simulink model "oving2"  (R2023a)
settings: Solver=ode1  StartTime=0.0  StopTime=25  FixedStep=0.01  RelTol=1e-9  AbsTol=1e-9
values from neighbouring files (symbols this model uses):
  a = input('Skriv inn tallet "a" mellom 0 og 10: ')    [kap2_matlab_kode.m]    (also in kap3_kode_for_alle_figurene.m = 3)
  b = input('Skriv inn tallet "b" mellom 0 og 10: ')    [kap2_matlab_kode.m]
  c = 3    [kap2_matlab_kode.m]    (also in kap3_kode_for_alle_figurene.m = 0.785398163397)
  d = 6.4    [kap2_matlab_kode.m]    (also in kap3_kode_for_alle_figurene.m = 4)
  f = int8(d)    [kap2_matlab_kode.m]    (also in kap3_kode_for_alle_figurene.m = sin(t); oving3_LL.m = 4.2)
  g = 5    [kap2_matlab_kode.m]
  h = 3    [kap2_matlab_kode.m]
  k = length(x)    [kap2_matlab_kode.m]    (also in kap3_kode_for_alle_figurene.m = 2; oving3_LL.m = 2)
  n = 7    [oving3_LL.m]
undefined symbols (not defined in the file or in its folder): i, j, l, m, o, p
libraries: simulink x16
settings Model: Creator=tormod  LastModifiedBy=redfox
settings DebuggingCC: UnconnectedInputMsg=warning  UnconnectedOutputMsg=warning  UnconnectedLineMsg=warning
settings ModelReferenceCC: EnableRefExpFcnMdlSchedulingChecks=on
settings RTWCC: DLArmComputeVersion=19.05

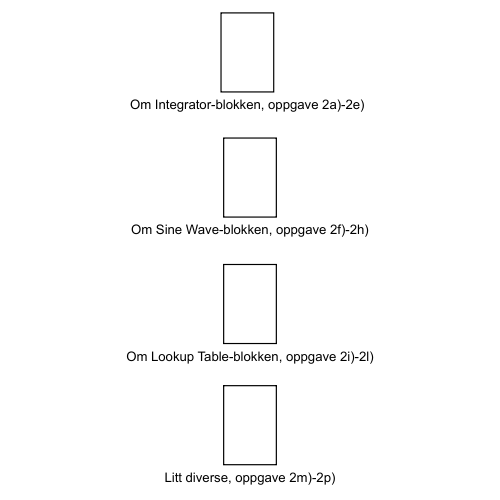
[thumbnail: Simulink's stored preview of the top-level diagram]
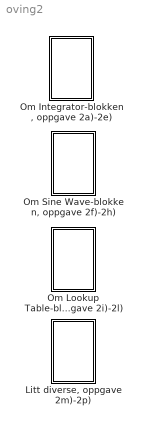
== system oving2 ==
  "Litt diverse, oppgave 2m)-2p)" : Subsystem
  "Om Integrator-blokken, oppgave 2a)-2e)" : Subsystem
  "Om Lookup Table-blokken, oppgave 2i)-2l)" : Subsystem
  "Om Sine Wave-blokken, oppgave 2f)-2h)" : Subsystem

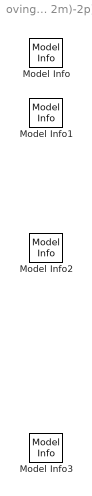
== system oving2/Litt diverse, oppgave 2m)-2p) ==
  Model Info : simulink/Model-Wide Utilities/Model Info  Frame=on  DisplayStringWithTags=m)  HorizontalTextAlignment=Center  LeftAlignmentValue=0.5
  Model Info1 : simulink/Model-Wide Utilities/Model Info  Frame=on  DisplayStringWithTags=n)  HorizontalTextAlignment=Center  LeftAlignmentValue=0.5
  Model Info2 : simulink/Model-Wide Utilities/Model Info  Frame=on  DisplayStringWithTags=o)  HorizontalTextAlignment=Center  LeftAlignmentValue=0.5
  Model Info3 : simulink/Model-Wide Utilities/Model Info  Frame=on  DisplayStringWithTags=p)  HorizontalTextAlignment=Center  LeftAlignmentValue=0.5

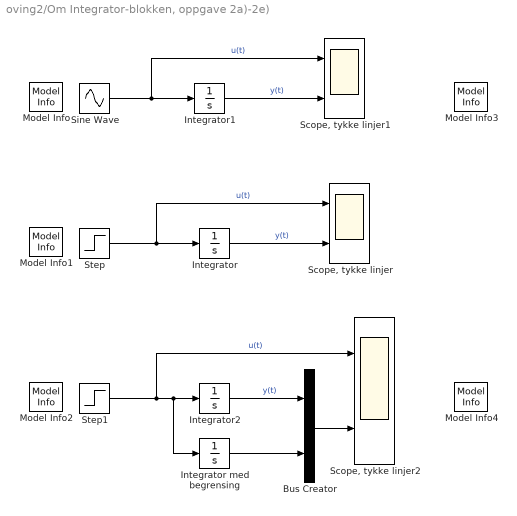
== system oving2/Om Integrator-blokken, oppgave 2a)-2e) ==
  Bus Creator : BusCreator  Inputs=2
  Integrator : Integrator  InitialCondition=-20
      settings: AttributesFormatString=IC = %<InitialCondition>
  Integrator med begrensing : Integrator  InitialCondition=-20  LimitOutput=on  UpperSaturationLimit=30
      settings: AttributesFormatString=|
      | IC = %<InitialCondition>
      | Max = %<UpperSaturationLimit>
      | Min = %<LowerSaturationLimit>
  Integrator1 : Integrator
      settings: AttributesFormatString=IC = %<InitialCondition>
  Integrator2 : Integrator  InitialCondition=-20
      settings: AttributesFormatString=IC = %<InitialCondition>
  Model Info : simulink/Model-Wide Utilities/Model Info  Frame=on  DisplayStringWithTags=a)  HorizontalTextAlignment=Center  LeftAlignmentValue=0.5
  Model Info1 : simulink/Model-Wide Utilities/Model Info  Frame=on  DisplayStringWithTags=b)  HorizontalTextAlignment=Center  LeftAlignmentValue=0.5
  Model Info2 : simulink/Model-Wide Utilities/Model Info  Frame=on  DisplayStringWithTags=c)  HorizontalTextAlignment=Center  LeftAlignmentValue=0.5
  Model Info3 : simulink/Model-Wide Utilities/Model Info  Frame=on  DisplayStringWithTags=d)  HorizontalTextAlignment=Center  LeftAlignmentValue=0.5
  Model Info4 : simulink/Model-Wide Utilities/Model Info  Frame=on  DisplayStringWithTags=e)  HorizontalTextAlignment=Center  LeftAlignmentValue=0.5
  "Scope, tykke linjer" : Scope  NumInputPorts=2
  "Scope, tykke linjer1" : Scope  NumInputPorts=2
  "Scope, tykke linjer2" : Scope  NumInputPorts=2
  Sine Wave : Sin  Amplitude=2  Frequency=5  SampleTime=0
      settings: AttributesFormatString=u(t) = %<Amplitude> sin(%<Frequency>t + %<Phase>) + %<Bias>
  Step : Step  Time=5  After=4  SampleTime=0
      settings: AttributesFormatString=|
      | u(t) = %<Before> for t < %<Time>s
      |       = %<After> for t > %<Time>s
  Step1 : Step  Time=5  After=4  SampleTime=0
      settings: AttributesFormatString=|
      | u(t) = %<Before> for t < %<Time>s
      |       = %<After> for t > %<Time>s
  wires:
  Step/1 -> "Scope, tykke linjer"/1, Integrator/1  "u(t)"
  Integrator/1 -> "Scope, tykke linjer"/2  "y(t)"
  Integrator1/1 -> "Scope, tykke linjer1"/2  "y(t)"
  Sine Wave/1 -> "Scope, tykke linjer1"/1, Integrator1/1  "u(t)"
  Integrator2/1 -> Bus Creator/1  "y(t)"
  Step1/1 -> "Scope, tykke linjer2"/1, Integrator med begrensing/1, Integrator2/1  "u(t)"
  Bus Creator/1 -> "Scope, tykke linjer2"/2
  Integrator med begrensing/1 -> Bus Creator/2

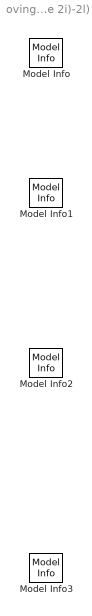
== system oving2/Om Lookup Table-blokken, oppgave 2i)-2l) ==
  Model Info : simulink/Model-Wide Utilities/Model Info  Frame=on  DisplayStringWithTags=i)  HorizontalTextAlignment=Center  LeftAlignmentValue=0.5
  Model Info1 : simulink/Model-Wide Utilities/Model Info  Frame=on  DisplayStringWithTags=j)  HorizontalTextAlignment=Center  LeftAlignmentValue=0.5
  Model Info2 : simulink/Model-Wide Utilities/Model Info  Frame=on  DisplayStringWithTags=k)  HorizontalTextAlignment=Center  LeftAlignmentValue=0.5
  Model Info3 : simulink/Model-Wide Utilities/Model Info  Frame=on  DisplayStringWithTags=l)  HorizontalTextAlignment=Center  LeftAlignmentValue=0.5

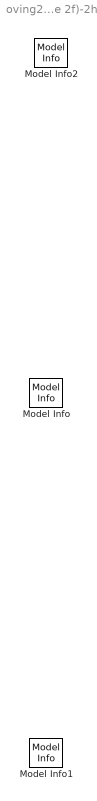
== system oving2/Om Sine Wave-blokken, oppgave 2f)-2h) ==
  Model Info : simulink/Model-Wide Utilities/Model Info  Frame=on  DisplayStringWithTags=g)  HorizontalTextAlignment=Center  LeftAlignmentValue=0.5
  Model Info1 : simulink/Model-Wide Utilities/Model Info  Frame=on  DisplayStringWithTags=h)  HorizontalTextAlignment=Center  LeftAlignmentValue=0.5
  Model Info2 : simulink/Model-Wide Utilities/Model Info  Frame=on  DisplayStringWithTags=f)  HorizontalTextAlignment=Center  LeftAlignmentValue=0.5
